simulink model "bcddevresinie3ecevirme"  (R2013a)
settings: Solver=ode45  StartTime=0.0  StopTime=10.0  RelTol=1e-3
settings Model: Creator=Lenovo  LastModifiedBy=Lenovo

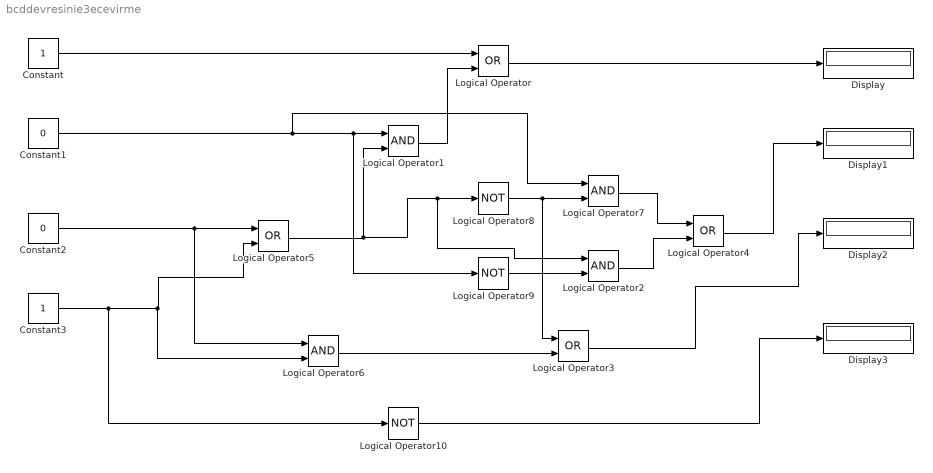
== system bcddevresinie3ecevirme ==
  Constant : Constant
  Constant1 : Constant  Value=0
  Constant2 : Constant  Value=0
  Constant3 : Constant
  Display{,1..3} (4 alike) : Display
  Logical Operator{,3..5} (4 alike) : Logic  Operator=OR  AllPortsSameDT=off  OutDataTypeStr=boolean
  Logical Operator{1..2,6..7} (4 alike) : Logic  AllPortsSameDT=off  OutDataTypeStr=boolean
  Logical Operator10 : Logic  Operator=NOT  AllPortsSameDT=off  OutDataTypeStr=boolean
  Logical Operator8 : Logic  Operator=NOT  AllPortsSameDT=off  OutDataTypeStr=boolean
  Logical Operator9 : Logic  Operator=NOT  AllPortsSameDT=off  OutDataTypeStr=boolean
  wires:
  Logical Operator4/1 -> Display1/1
  Logical Operator3/1 -> Display2/1
  Logical Operator10/1 -> Display3/1
  Logical Operator/1 -> Display/1
  Logical Operator9/1 -> Logical Operator2/2
  Logical Operator8/1 -> Logical Operator3/1, Logical Operator7/2
  Logical Operator1/1 -> Logical Operator/2
  Logical Operator6/1 -> Logical Operator3/2
  Logical Operator7/1 -> Logical Operator4/1
  Logical Operator2/1 -> Logical Operator4/2
  Constant/1 -> Logical Operator/1
  Constant2/1 -> Logical Operator6/1, Logical Operator5/1
  Constant3/1 -> Logical Operator10/1, Logical Operator6/2, Logical Operator5/2
  Logical Operator5/1 -> Logical Operator2/1, Logical Operator8/1, Logical Operator1/2
  Constant1/1 -> Logical Operator7/1, Logical Operator9/1, Logical Operator1/1
